simulink model "step6_3_controller_PID"  (R2022b)
settings: Solver=FixedStepAuto  StartTime=0.0  StopTime=RunTime  FixedStep=time_step  RelTol=1e-3
values from neighbouring files (symbols this model uses):
  A = [0 1 0 0 ... (first row only)    [linearize_script.m]    (also in step4_0_linearize_operating_point.m = double(A); step4_linearized_system.mat = [0 0.339319496362 0 -114.426616159 0 1 -102.612245897 0 221.; syms_test.m = double(A))
  B = [0 ... (first row only)    [linearize_script.m]    (also in step4_0_linearize_operating_point.m = double(B); step4_linearized_system.mat = [0 0 0 0 5076.90787281]; syms_test.m = double(B))
  C = [1 0 0 0 ... (first row only)    [linearize_script.m]    (also in matrixmaker_linearization.m = [b_1_0 - P_3 * theta_d_2 * sin(theta_2)  -P_3 * (theta_d_1 +; step4_0_linearize_operating_point.m = [1 0 0 0 0; step4_linearized_system.mat = [1  0  0  0  0; 0  0  1  0  0]; syms_test.m)
  D = zeros(2,1)    [linearize_script.m]    (also in step4_0_linearize_operating_point.m; step4_linearized_system.mat = [0 0]; syms_test.m)
  g1 = (m_1 * c_1_0 + m_2 * l_1) * g    [compare_ourmodel_with_others.m]    (also in step2_whitebox_beam.m; step4_0_linearize_operating_point.m; step5_observor_design.m; step6_1_controller_feedback.m)
  g2 = m_2 * c_2_0 * g    [compare_ourmodel_with_others.m]    (also in step2_whitebox_beam.m; step4_0_linearize_operating_point.m; step5_observor_design.m; step6_1_controller_feedback.m)
  P1 = m_1 * c_1_0 * c_1_0 + m_2 * l_1 * l_1 + I_1_0    [compare_ourmodel_with_others.m]    (also in script_for_test.m = P2(1:L/2+1); step2_whitebox_beam.m; step4_0_linearize_operating_point.m; step5_observor_design.m)
  P2 = m_2 * c_2_0 * c_2_0 + I_2_0    [compare_ourmodel_with_others.m]    (also in script_for_test.m = abs(Y/L); step2_whitebox_beam.m; step4_0_linearize_operating_point.m; step5_observor_design.m)
  P3 = m_2 * l_1 * c_2_0    [compare_ourmodel_with_others.m]    (also in step2_whitebox_beam.m; step4_0_linearize_operating_point.m; step5_observor_design.m; step6_1_controller_feedback.m)
  params = [9.81, 0.1, 0.1, 0.125, 0.05, -0.0300000121036330, 0.0813451968350115, 0.1000000000017210, 2.00882387117299e-05, 10.27570530021582, 2.78577414601457e-05, 65.9998023466922, 0.01300000000002200]    [compare_ourmodel_with_others.m]    (also in linearization.m = params_hat; matrixmaker_linearization.m = [-0.001, 0.077, 0.2, 0.00004, 20.684, 0.0004, 15, 0.03]; params.mat = [9.81 0.1 0.1 0.125 0.046955 -0.032 0.04609 0.0888 9.9e-05 6; sss.m = [9.81, 0.1, 0.1, 0.125, 0.04824, -0.041443, .0607558, 0.1154)
  theta_1_0 = pi    (= 3.14159265359)    [hwinit.m]    (also in hwinit_raw.m; step4_0_linearize_operating_point.m; step5_observor_design.m = x_op(1); step6_1_controller_feedback.m = x_op(1))
  theta_2_0 = 0    [hwinit.m]    (also in hwinit_raw.m; step4_0_linearize_operating_point.m; step5_observor_design.m = x_op(3); step6_1_controller_feedback.m = x_op(3))
  x_op_relative = [0; 0; 0; 0; 0]    [step5_observor_design.m]    (also in step6_1_controller_feedback.m)
libraries: slpidlib x4
settings Model: Creator=annel  LastModifiedBy=97083

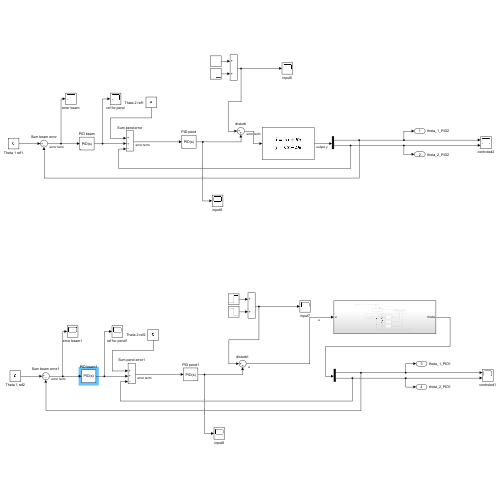
[thumbnail: Simulink's stored preview of the top-level diagram]
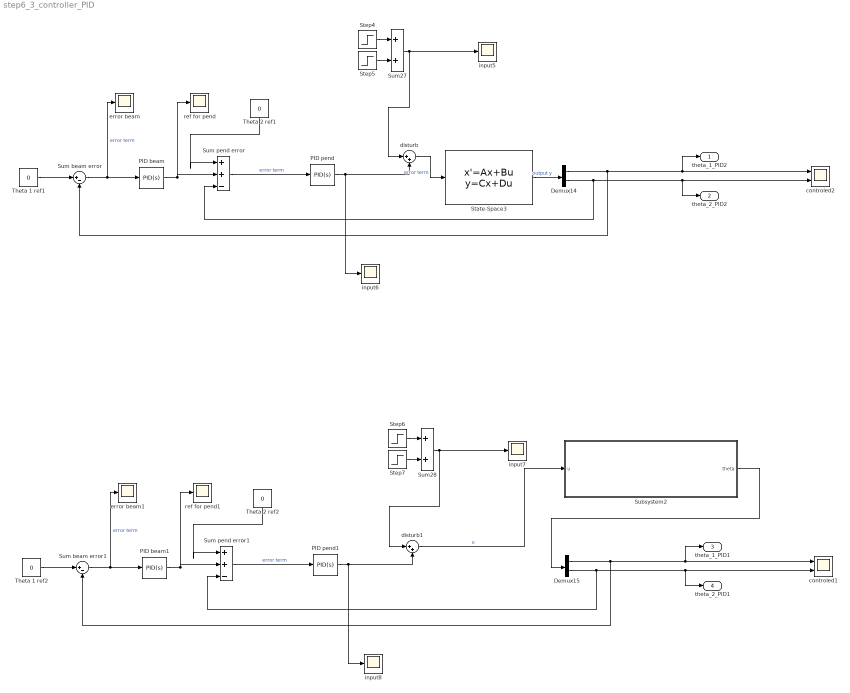
== system step6_3_controller_PID ==
  Demux14 : Demux  Outputs=2
  Demux15 : Demux  Outputs=2
  PID beam : slpidlib/PID Controller  Controller=PID  Form=Parallel  TimeDomain=Continuous-time  UseExternalTs=off  SampleTime=-1  IntegratorMethod=Forward Euler  FilterMethod=Forward Euler  ControllerParametersSource=internal  P=0.5  I=-0.1  UseKiTs=off  D=-0.079  N=0.05  UseFilter=on  TunerSelectOption=Transfer Function Based (PID Tuner App)  InitialConditionSource=internal  InitialConditionForIntegrator=0  InitialConditionForFilter=0  DifferentiatorICPrevScaledInput=0  ExternalReset=none  TrackingMode=off  Kt=1  LimitOutput=off  SatLimitsSource=internal  UpperSaturationLimit=inf  LowerSaturationLimit=-inf  LinearizeAsGain=on  AntiWindupMode=none  Kb=1  LimitIntegrator=off  UpperIntegratorSaturationLimit=inf  LowerIntegratorSaturationLimit=-inf  POutMin=[]  POutMax=[]  IOutMin=[]  IOutMax=[]  DOutMin=[]  DOutMax=[]  NOutMin=[]  NOutMax=[]  SumOutMin=[]  SumOutMax=[]  SaturationOutMin=[]  SaturationOutMax=[]  PParamMin=[]  PParamMax=[]  IParamMin=[]  IParamMax=[]  DParamMin=[]  DParamMax=[]  NParamMin=[]  NParamMax=[]  KbParamMin=[]  KbParamMax=[]  KtParamMin=[]  KtParamMax=[]  KbOutMin=[]  KbOutMax=[]  KtOutMin=[]  KtOutMax=[]  IntegratorOutMin=[]  IntegratorOutMax=[]  FilterOutMin=[]  FilterOutMax=[]  SumI1OutMin=[]  SumI1OutMax=[]  SumI2OutMin=[]  SumI2OutMax=[]  SumI3OutMin=[]  SumI3OutMax=[]  SumI4OutMin=[]  SumI4OutMax=[]  SumDOutMin=[]  SumDOutMax=[]  DifferentiatorOutMin=[]  DifferentiatorOutMax=[]  FilterDiffOutCoefMin=[]  FilterDiffOutCoefMax=[]  ReciprocalOutMin=[]  ReciprocalOutMax=[]  SumDenOutMin=[]  SumDenOutMax=[]  SumNumOutMin=[]  SumNumOutMax=[]  DivideOutMin=[]  DivideOutMax=[]  UdiffTsProdOutMin=[]  UdiffTsProdOutMax=[]  NTsProdOutMin=[]  NTsProdOutMax=[]  UintegralTsProdOutMin=[]  UintegralTsProdOutMax=[]  UngainTsProdOutMin=[]  UngainTsProdOutMax=[]  ClampingZeroOutDataTypeStr=Inherit: Inherit via back propagation  ClampingZeroOutMin=[]  ClampingZeroOutMax=[]  FilterDenConstantOutDataTypeStr=Inherit: Inherit via back propagation  FilterDenConstantOutMin=[]  FilterDenConstantOutMax=[]  PCopyOutDataTypeStr=Inherit: Inherit via back propagation  PCopyOutMin=[]  PCopyOutMax=[]  NCopyOutDataTypeStr=Inherit: Inherit via back propagation  NCopyOutMin=[]  NCopyOutMax=[]  IntegratorContinuousStateAttributes=''  IntegratorStateMustResolveToSignalObject=off  IntegratorRTWStateStorageClass=Auto  FilterContinuousStateAttributes=''  FilterStateMustResolveToSignalObject=off  FilterRTWStateStorageClass=Auto  ParallelPVariant=InternalParameters  IdealPVariant=Disabled  IVariant=InternalParameters  DVariant=InternalParameters  IntegratorVariant=Continuous  SatVariant=Disabled  AWVariant=Passthrough  PCopyVariant=Disabled  TRVariant=Disabled  FdbkBlocksVariant=Forward  IdealPFdbkVariant=Disabled  SatFdbkVariant=Disabled  DerivativeFilterVariant=ContFilter  NVariant=InternalParameters  NCopyVariant=Disabled  FilterICVariant=InternalICsFilter  IntegratorICVariant=InternalICs  ExternalResetVariant=Disabled  TRSumVariant=Passthrough  SumFdbkVariant=Disabled  SumVariant=Sum_PID  TsampFilterVariant=InternalTs  TsampNgainVariant=Passthrough  TsampIntegralVariant=Passthrough  ExternalSaturationOutDataTypeStr=Inherit: Same as second input
  PID beam1 : slpidlib/PID Controller  Controller=PID  Form=Parallel  TimeDomain=Continuous-time  UseExternalTs=off  SampleTime=-1  IntegratorMethod=Forward Euler  FilterMethod=Forward Euler  ControllerParametersSource=internal  P=0.005  I=-0.1  UseKiTs=off  D=-0.079  N=0.05  UseFilter=on  TunerSelectOption=Transfer Function Based (PID Tuner App)  InitialConditionSource=internal  InitialConditionForIntegrator=0  InitialConditionForFilter=0  DifferentiatorICPrevScaledInput=0  ExternalReset=none  TrackingMode=off  Kt=1  LimitOutput=off  SatLimitsSource=internal  UpperSaturationLimit=inf  LowerSaturationLimit=-inf  LinearizeAsGain=on  AntiWindupMode=none  Kb=1  LimitIntegrator=off  UpperIntegratorSaturationLimit=inf  LowerIntegratorSaturationLimit=-inf  POutMin=[]  POutMax=[]  IOutMin=[]  IOutMax=[]  DOutMin=[]  DOutMax=[]  NOutMin=[]  NOutMax=[]  SumOutMin=[]  SumOutMax=[]  SaturationOutMin=[]  SaturationOutMax=[]  PParamMin=[]  PParamMax=[]  IParamMin=[]  IParamMax=[]  DParamMin=[]  DParamMax=[]  NParamMin=[]  NParamMax=[]  KbParamMin=[]  KbParamMax=[]  KtParamMin=[]  KtParamMax=[]  KbOutMin=[]  KbOutMax=[]  KtOutMin=[]  KtOutMax=[]  IntegratorOutMin=[]  IntegratorOutMax=[]  FilterOutMin=[]  FilterOutMax=[]  SumI1OutMin=[]  SumI1OutMax=[]  SumI2OutMin=[]  SumI2OutMax=[]  SumI3OutMin=[]  SumI3OutMax=[]  SumI4OutMin=[]  SumI4OutMax=[]  SumDOutMin=[]  SumDOutMax=[]  DifferentiatorOutMin=[]  DifferentiatorOutMax=[]  FilterDiffOutCoefMin=[]  FilterDiffOutCoefMax=[]  ReciprocalOutMin=[]  ReciprocalOutMax=[]  SumDenOutMin=[]  SumDenOutMax=[]  SumNumOutMin=[]  SumNumOutMax=[]  DivideOutMin=[]  DivideOutMax=[]  UdiffTsProdOutMin=[]  UdiffTsProdOutMax=[]  NTsProdOutMin=[]  NTsProdOutMax=[]  UintegralTsProdOutMin=[]  UintegralTsProdOutMax=[]  UngainTsProdOutMin=[]  UngainTsProdOutMax=[]  ClampingZeroOutDataTypeStr=Inherit: Inherit via back propagation  ClampingZeroOutMin=[]  ClampingZeroOutMax=[]  FilterDenConstantOutDataTypeStr=Inherit: Inherit via back propagation  FilterDenConstantOutMin=[]  FilterDenConstantOutMax=[]  PCopyOutDataTypeStr=Inherit: Inherit via back propagation  PCopyOutMin=[]  PCopyOutMax=[]  NCopyOutDataTypeStr=Inherit: Inherit via back propagation  NCopyOutMin=[]  NCopyOutMax=[]  IntegratorContinuousStateAttributes=''  IntegratorStateMustResolveToSignalObject=off  IntegratorRTWStateStorageClass=Auto  FilterContinuousStateAttributes=''  FilterStateMustResolveToSignalObject=off  FilterRTWStateStorageClass=Auto  ParallelPVariant=InternalParameters  IdealPVariant=Disabled  IVariant=InternalParameters  DVariant=InternalParameters  IntegratorVariant=Continuous  SatVariant=Disabled  AWVariant=Passthrough  PCopyVariant=Disabled  TRVariant=Disabled  FdbkBlocksVariant=Forward  IdealPFdbkVariant=Disabled  SatFdbkVariant=Disabled  DerivativeFilterVariant=ContFilter  NVariant=InternalParameters  NCopyVariant=Disabled  FilterICVariant=InternalICsFilter  IntegratorICVariant=InternalICs  ExternalResetVariant=Disabled  TRSumVariant=Passthrough  SumFdbkVariant=Disabled  SumVariant=Sum_PID  TsampFilterVariant=InternalTs  TsampNgainVariant=Passthrough  TsampIntegralVariant=Passthrough  ExternalSaturationOutDataTypeStr=Inherit: Same as second input
  PID pend : slpidlib/PID Controller  Controller=PID  Form=Parallel  TimeDomain=Continuous-time  UseExternalTs=off  SampleTime=-1  IntegratorMethod=Forward Euler  FilterMethod=Forward Euler  ControllerParametersSource=internal  P=3  I=0.1  UseKiTs=off  D=0.0083  N=3  UseFilter=on  TunerSelectOption=Transfer Function Based (PID Tuner App)  InitialConditionSource=internal  InitialConditionForIntegrator=0  InitialConditionForFilter=0  DifferentiatorICPrevScaledInput=0  ExternalReset=none  TrackingMode=off  Kt=1  LimitOutput=off  SatLimitsSource=internal  UpperSaturationLimit=inf  LowerSaturationLimit=-inf  LinearizeAsGain=on  AntiWindupMode=none  Kb=1  LimitIntegrator=off  UpperIntegratorSaturationLimit=inf  LowerIntegratorSaturationLimit=-inf  POutMin=[]  POutMax=[]  IOutMin=[]  IOutMax=[]  DOutMin=[]  DOutMax=[]  NOutMin=[]  NOutMax=[]  SumOutMin=[]  SumOutMax=[]  SaturationOutMin=[]  SaturationOutMax=[]  PParamMin=[]  PParamMax=[]  IParamMin=[]  IParamMax=[]  DParamMin=[]  DParamMax=[]  NParamMin=[]  NParamMax=[]  KbParamMin=[]  KbParamMax=[]  KtParamMin=[]  KtParamMax=[]  KbOutMin=[]  KbOutMax=[]  KtOutMin=[]  KtOutMax=[]  IntegratorOutMin=[]  IntegratorOutMax=[]  FilterOutMin=[]  FilterOutMax=[]  SumI1OutMin=[]  SumI1OutMax=[]  SumI2OutMin=[]  SumI2OutMax=[]  SumI3OutMin=[]  SumI3OutMax=[]  SumI4OutMin=[]  SumI4OutMax=[]  SumDOutMin=[]  SumDOutMax=[]  DifferentiatorOutMin=[]  DifferentiatorOutMax=[]  FilterDiffOutCoefMin=[]  FilterDiffOutCoefMax=[]  ReciprocalOutMin=[]  ReciprocalOutMax=[]  SumDenOutMin=[]  SumDenOutMax=[]  SumNumOutMin=[]  SumNumOutMax=[]  DivideOutMin=[]  DivideOutMax=[]  UdiffTsProdOutMin=[]  UdiffTsProdOutMax=[]  NTsProdOutMin=[]  NTsProdOutMax=[]  UintegralTsProdOutMin=[]  UintegralTsProdOutMax=[]  UngainTsProdOutMin=[]  UngainTsProdOutMax=[]  ClampingZeroOutDataTypeStr=Inherit: Inherit via back propagation  ClampingZeroOutMin=[]  ClampingZeroOutMax=[]  FilterDenConstantOutDataTypeStr=Inherit: Inherit via back propagation  FilterDenConstantOutMin=[]  FilterDenConstantOutMax=[]  PCopyOutDataTypeStr=Inherit: Inherit via back propagation  PCopyOutMin=[]  PCopyOutMax=[]  NCopyOutDataTypeStr=Inherit: Inherit via back propagation  NCopyOutMin=[]  NCopyOutMax=[]  IntegratorContinuousStateAttributes=''  IntegratorStateMustResolveToSignalObject=off  IntegratorRTWStateStorageClass=Auto  FilterContinuousStateAttributes=''  FilterStateMustResolveToSignalObject=off  FilterRTWStateStorageClass=Auto  ParallelPVariant=InternalParameters  IdealPVariant=Disabled  IVariant=InternalParameters  DVariant=InternalParameters  IntegratorVariant=Continuous  SatVariant=Disabled  AWVariant=Passthrough  PCopyVariant=Disabled  TRVariant=Disabled  FdbkBlocksVariant=Forward  IdealPFdbkVariant=Disabled  SatFdbkVariant=Disabled  DerivativeFilterVariant=ContFilter  NVariant=InternalParameters  NCopyVariant=Disabled  FilterICVariant=InternalICsFilter  IntegratorICVariant=InternalICs  ExternalResetVariant=Disabled  TRSumVariant=Passthrough  SumFdbkVariant=Disabled  SumVariant=Sum_PID  TsampFilterVariant=InternalTs  TsampNgainVariant=Passthrough  TsampIntegralVariant=Passthrough  ExternalSaturationOutDataTypeStr=Inherit: Same as second input
  PID pend1 : slpidlib/PID Controller  Controller=PID  Form=Parallel  TimeDomain=Continuous-time  UseExternalTs=off  SampleTime=-1  IntegratorMethod=Forward Euler  FilterMethod=Forward Euler  ControllerParametersSource=internal  P=0.05  I=0.1  UseKiTs=off  D=0.0083  N=3  UseFilter=on  TunerSelectOption=Transfer Function Based (PID Tuner App)  InitialConditionSource=internal  InitialConditionForIntegrator=0  InitialConditionForFilter=0  DifferentiatorICPrevScaledInput=0  ExternalReset=none  TrackingMode=off  Kt=1  LimitOutput=off  SatLimitsSource=internal  UpperSaturationLimit=inf  LowerSaturationLimit=-inf  LinearizeAsGain=on  AntiWindupMode=none  Kb=1  LimitIntegrator=off  UpperIntegratorSaturationLimit=inf  LowerIntegratorSaturationLimit=-inf  POutMin=[]  POutMax=[]  IOutMin=[]  IOutMax=[]  DOutMin=[]  DOutMax=[]  NOutMin=[]  NOutMax=[]  SumOutMin=[]  SumOutMax=[]  SaturationOutMin=[]  SaturationOutMax=[]  PParamMin=[]  PParamMax=[]  IParamMin=[]  IParamMax=[]  DParamMin=[]  DParamMax=[]  NParamMin=[]  NParamMax=[]  KbParamMin=[]  KbParamMax=[]  KtParamMin=[]  KtParamMax=[]  KbOutMin=[]  KbOutMax=[]  KtOutMin=[]  KtOutMax=[]  IntegratorOutMin=[]  IntegratorOutMax=[]  FilterOutMin=[]  FilterOutMax=[]  SumI1OutMin=[]  SumI1OutMax=[]  SumI2OutMin=[]  SumI2OutMax=[]  SumI3OutMin=[]  SumI3OutMax=[]  SumI4OutMin=[]  SumI4OutMax=[]  SumDOutMin=[]  SumDOutMax=[]  DifferentiatorOutMin=[]  DifferentiatorOutMax=[]  FilterDiffOutCoefMin=[]  FilterDiffOutCoefMax=[]  ReciprocalOutMin=[]  ReciprocalOutMax=[]  SumDenOutMin=[]  SumDenOutMax=[]  SumNumOutMin=[]  SumNumOutMax=[]  DivideOutMin=[]  DivideOutMax=[]  UdiffTsProdOutMin=[]  UdiffTsProdOutMax=[]  NTsProdOutMin=[]  NTsProdOutMax=[]  UintegralTsProdOutMin=[]  UintegralTsProdOutMax=[]  UngainTsProdOutMin=[]  UngainTsProdOutMax=[]  ClampingZeroOutDataTypeStr=Inherit: Inherit via back propagation  ClampingZeroOutMin=[]  ClampingZeroOutMax=[]  FilterDenConstantOutDataTypeStr=Inherit: Inherit via back propagation  FilterDenConstantOutMin=[]  FilterDenConstantOutMax=[]  PCopyOutDataTypeStr=Inherit: Inherit via back propagation  PCopyOutMin=[]  PCopyOutMax=[]  NCopyOutDataTypeStr=Inherit: Inherit via back propagation  NCopyOutMin=[]  NCopyOutMax=[]  IntegratorContinuousStateAttributes=''  IntegratorStateMustResolveToSignalObject=off  IntegratorRTWStateStorageClass=Auto  FilterContinuousStateAttributes=''  FilterStateMustResolveToSignalObject=off  FilterRTWStateStorageClass=Auto  ParallelPVariant=InternalParameters  IdealPVariant=Disabled  IVariant=InternalParameters  DVariant=InternalParameters  IntegratorVariant=Continuous  SatVariant=Disabled  AWVariant=Passthrough  PCopyVariant=Disabled  TRVariant=Disabled  FdbkBlocksVariant=Forward  IdealPFdbkVariant=Disabled  SatFdbkVariant=Disabled  DerivativeFilterVariant=ContFilter  NVariant=InternalParameters  NCopyVariant=Disabled  FilterICVariant=InternalICsFilter  IntegratorICVariant=InternalICs  ExternalResetVariant=Disabled  TRSumVariant=Passthrough  SumFdbkVariant=Disabled  SumVariant=Sum_PID  TsampFilterVariant=InternalTs  TsampNgainVariant=Passthrough  TsampIntegralVariant=Passthrough  ExternalSaturationOutDataTypeStr=Inherit: Same as second input
  State-Space3 : StateSpace  A=A  B=B  C=C  D=D  InitialCondition=x_op_relative
  Step4 : Step
  Step5 : Step  Time=1.1  After=-1
  Step6 : Step  After=0.3
  Step7 : Step  Time=1.1  After=-0.3
  Subsystem2 : Subsystem
  Sum beam error : Sum  Inputs=|+-
  Sum beam error1 : Sum  Inputs=|+-
  Sum pend error : Sum  Inputs=|++-
  Sum pend error1 : Sum  Inputs=|++-
  Sum27 : Sum
  Sum28 : Sum
  Theta 1 ref1 : Constant  Value=0
  Theta 1 ref2 : Constant  Value=0
  Theta 2 ref1 : Constant  Value=0
  Theta 2 ref2 : Constant  Value=0
  controled1 : Scope  NumInputPorts=2
  controled2 : Scope  NumInputPorts=2
  disturb : Sum  Inputs=|++
  disturb1 : Sum  Inputs=|++
  error beam : Scope
  error beam1 : Scope
  input{5..8} (4 alike) : Scope
  ref for pend : Scope
  ref for pend1 : Scope
  theta_1_PID2 : Outport
  theta_2_PID2 : Outport  Port=2
  theta_1_PID1 : Outport  Port=3
  theta_2_PID1 : Outport  Port=4
  wires:
  Sum27/1 -> input5/1, disturb/1
  Step5/1 -> Sum27/2
  disturb/1 -> State-Space3/1  "error term"
  Theta 2 ref1/1 -> Sum pend error/1
  PID pend/1 -> input6/1, disturb/2
  Step4/1 -> Sum27/1
  State-Space3/1 -> Demux14/1  "output y"
  Demux14/2 -> Sum pend error/3, theta_2_PID2/1, controled2/2
  Demux14/1 -> theta_1_PID2/1, controled2/1, Sum beam error/2
  Sum pend error/1 -> PID pend/1  "error term"
  Sum beam error/1 -> error beam/1, PID beam/1  "error term"
  PID beam/1 -> ref for pend/1, Sum pend error/2
  Theta 1 ref1/1 -> Sum beam error/1
  Theta 1 ref2/1 -> Sum beam error1/1
  PID beam1/1 -> ref for pend1/1, Sum pend error1/2
  Sum pend error1/1 -> PID pend1/1  "error term"
  Demux15/2 -> Sum pend error1/3, theta_2_PID1/1, controled1/2
  Demux15/1 -> theta_1_PID1/1, controled1/1, Sum beam error1/2
  PID pend1/1 -> input8/1, disturb1/2
  Theta 2 ref2/1 -> Sum pend error1/1
  Sum beam error1/1 -> error beam1/1, PID beam1/1  "error term"
  disturb1/1 -> Subsystem2/1(u)  "u"
  Subsystem2/1(theta) -> Demux15/1
  Step6/1 -> Sum28/1
  Step7/1 -> Sum28/2
  Sum28/1 -> disturb1/1, input7/1

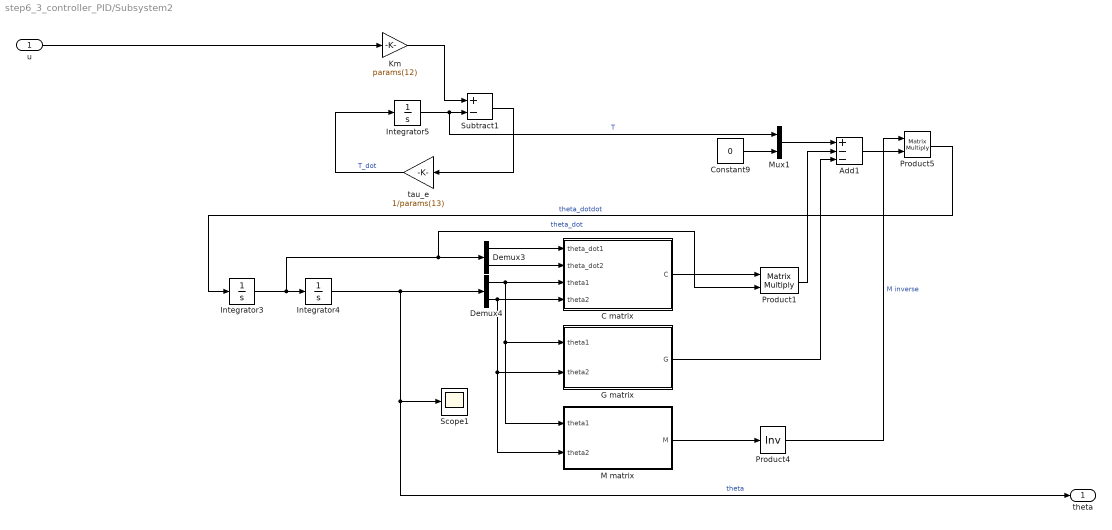
== system step6_3_controller_PID/Subsystem2 ==
  u : Inport
  Add1 : Sum  Inputs=+--
  C matrix : MATLAB Function  TreatAsAtomicUnit=on
  Constant9 : Constant  Value=0
  Demux3 : Demux  Outputs=2
  Demux4 : Demux  Outputs=2
  G matrix : MATLAB Function  TreatAsAtomicUnit=on
  Integrator3 : Integrator
  Integrator4 : Integrator  InitialCondition=[theta_1_0, theta_2_0]
  Integrator5 : Integrator
  Km : Gain  Gain=params(12)
  M matrix : MATLAB Function  TreatAsAtomicUnit=on
  Mux1 : Mux  Inputs=2
  Product1 : Product  Inputs=**  Multiplication=Matrix(*)
  Product4 : Product  Inputs=/  Multiplication=Matrix(*)
  Product5 : Product  Inputs=**  Multiplication=Matrix(*)
  Scope1 : Scope
  Subtract1 : Sum  Inputs=+-
  tau_e : Gain  Gain=1/params(13)
  theta : Outport
  wires:
  Demux4/1 -> M matrix/1(theta1), G matrix/1(theta1), C matrix/3(theta1)
  tau_e/1 -> Integrator5/1  "T_dot"
  Constant9/1 -> Mux1/2
  Demux3/1 -> C matrix/1(theta_dot1)
  Add1/1 -> Product5/2
  Subtract1/1 -> tau_e/1
  G matrix/1(G) -> Add1/3
  Integrator3/1 -> Product1/2, Demux3/1, Integrator4/1  "theta_dot"
  C matrix/1(C) -> Product1/1
  Mux1/1 -> Add1/1
  Integrator5/1 -> Mux1/1, Subtract1/2  "T"
  u/1 -> Km/1
  Product5/1 -> Integrator3/1  "theta_dotdot"
  Demux3/2 -> C matrix/2(theta_dot2)
  Integrator4/1 -> Demux4/1, theta/1, Scope1/1  "theta"
  M matrix/1(M) -> Product4/1
  Demux4/2 -> M matrix/2(theta2), G matrix/2(theta2), C matrix/4(theta2)
  Product4/1 -> Product5/1  "M inverse"
  Product1/1 -> Add1/2
  Km/1 -> Subtract1/1

== matlab function step6_3_controller_PID/Subsystem2/C matrix ==
  data: theta_dot1 input; theta_dot2 input; theta1 input; theta2 input; C output; params parameter; P3 parameter
function C = C(theta_dot1, theta_dot2, theta1, theta2, params, P3)
c00 = params(10) - P3 * theta_dot2 * sin(theta2);
c01 = -P3 * (theta_dot1 + theta_dot2) * sin(theta2);
c10 = P3 * theta_dot1 * sin(theta2);
c11 = params(11);

C = [c00 c01;
     c10 c11];

== matlab function step6_3_controller_PID/Subsystem2/G matrix ==
  data: theta1 input; theta2 input; G output; g1 parameter; g2 parameter
function G = G(theta1, theta2, g1, g2)
G00 = -g1 * sin(theta1) - g2 * sin(theta1 + theta2);
G01 = -g2 * sin(theta1 + theta2);

G = [G00 G01];

== matlab function step6_3_controller_PID/Subsystem2/M matrix ==
  data: theta1 input; theta2 input; M output; P1 parameter; P2 parameter; P3 parameter
function M = fcn(theta1, theta2, P1, P2, P3)
M00 = P1 + P2 + 2 * P3 * cos(theta2);
M01 = P2 + P3 * cos(theta2);
M10 = M01;
M11 = P2;

M = [M00 M01;
     M10 M11];
